simulink model "MotorModelDiscrete"  (R2019b)
settings: Solver=FixedStepAuto  StartTime=0.0  StopTime=8  FixedStep=Ts  RelTol=1e-3
undefined symbols (not defined in the file or in its folder): Discrete, motor, sensitivity_arduino, sigbuilder_block, Time, Ts
libraries: simulink x1, ctrlSharedLib x1, cstblocks x1, dspstat3 x1
settings Model: EnablePacing=on  Creator=miche  LastModifiedBy=AndreaCalegari

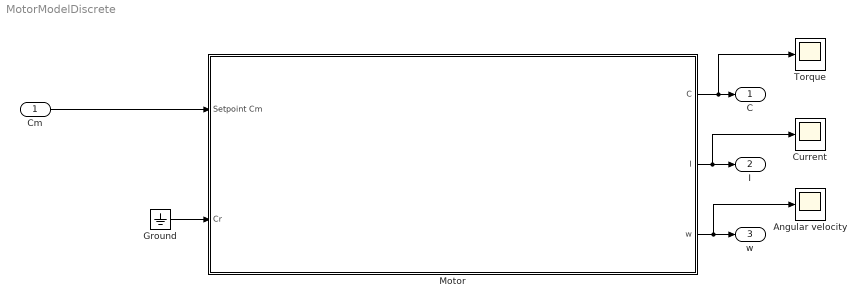
== system MotorModelDiscrete ==
  Cm : Inport
  Angular velocity : Scope
  Current : Scope
  Ground : Ground
  "Motor " : Subsystem
  Torque : Scope
  C : Outport
  I : Outport  Port=2
  w : Outport  Port=3
  wires:
  "Motor "/1("C ") -> Torque/1, C/1
  "Motor "/2("I ") -> Current/1, I/1
  "Motor "/3(w) -> Angular velocity/1, w/1
  Ground/1 -> "Motor "/2(Cr)
  Cm/1 -> "Motor "/1(Setpoint Cm)

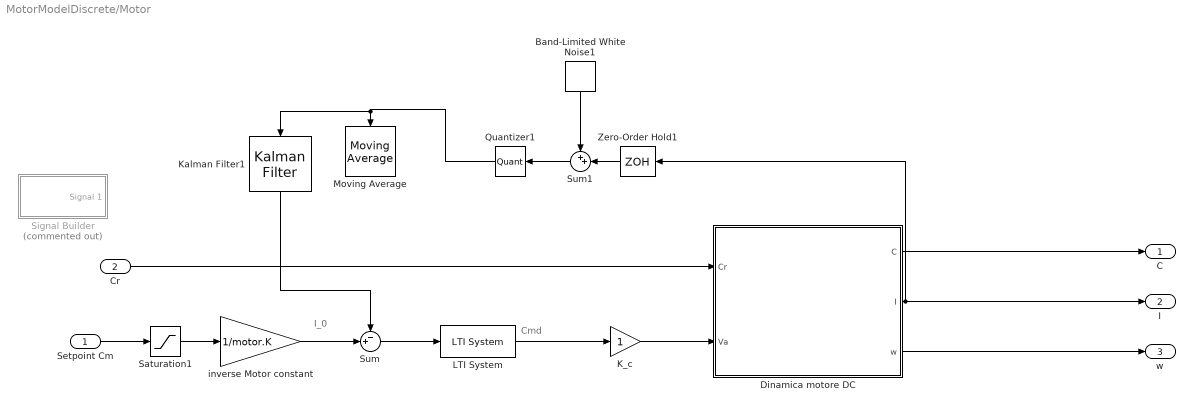
== system MotorModelDiscrete/Motor  ==
  note: Cmd
  note: I_0
  Setpoint Cm : Inport
  Cr : Inport  Port=2
  Band-Limited White Noise1 : simulink/Sources/Band-Limited White Noise  Cov=[0.00000001]  Ts=0.001  seed=[23341]
  Dinamica motore DC : Subsystem
  K_c : Gain
  Kalman Filter1 : ctrlSharedLib/Kalman Filter  TimeDomain=Discrete-Time  UseCurrentEstimator=on  ModelSource=Individual A, B, C, D matrices  ModelSourceVariable=ss(0.95,1,1,0,1)  A=0.999  B=1  C=1  D=0  NumberOfStates=1  NumberOfInputs=1  NumberOfOutputs=1  InitialEstimateSource=Dialog  X0=0  P0=10  UseK=off  UseGH=off  NumberOfProcessNoiseInputs=1  G=1  TimeInvariantG=on  H=0  TimeInvariantH=on  Q=0.1  TimeInvariantQ=on  R=1  TimeInvariantR=on  N=0  TimeInvariantN=on  AddInputPort=off  AddEnablePort=off  OutputEstimatedY=off  OutputP=off  Ts=-1
      settings: SourceProductBaseCode=CT
  LTI System : cstblocks/LTI System  sys=currentClosedLoop.PI_regulator_discrete  IC=[]
  Moving Average : dspstat3/Moving Average  Method=Sliding window  ForgettingFactorPort=off  SpecifyWindowLength=on  WindowLength=200  ForgettingFactor=0.9  SimulateUsing=Code generation
  Quantizer1 : Quantizer  QuantizationInterval=1/sensitivity_arduino
  Saturation1 : Saturate  UpperLimit=motor.Cmax  LowerLimit=-motor.Cmax
  Signal Builder : Subsystem  Tag=STV Subsys  Commented=on  LoadFcn=sigbuilder_block('load');  StartFcn=sigbuilder_block('start');  StopFcn=sigbuilder_block('stop');  ClipboardFcn=sigbuilder_block('clipboard');  mask(Sigbuilder block){tuvar=[0:10]}
      mask help: Simulink:masks:SigbuilderBlock_MD
      mask init:
      | if ~strcmp(get_param(bdroot(gcbh),'SimulationStatus'),'stopped') tuvar = sigbuilder_block('maskInit'); end
      settings: CopyFcn=sigbuilder_block('copy');  DeleteFcn=sigbuilder_block('delete');  ModelCloseFcn=sigbuilder_block('modelClose');  PreSaveFcn=sigbuilder_block('preSave');  PauseFcn=sigbuilder_block('pause');  ContinueFcn=sigbuilder_block('continue');  NameChangeFcn=sigbuilder_block('namechange');  OpenFcn=sigbuilder_block('open',[440.25 156.75 544.5 355.5 ]);  CloseFcn=sigbuilder_block('close');
      mask Display: plot(0, 0, 100, 100,[2, 2, 32, 32, 2], [68, 8, 8, 68, 68],[32, 2], [38, 38], [32, 19, 2],[53, 60, 44], [32, 17, 17, 2],[16, 16, 31, 31]);txt = getActiveGroup(gcbh);text(2, 100, txt,'verticalAlignment', 'top');
  Sum : Sum  Inputs=-+|
  Sum1 : Sum  Inputs=++|
  Zero-Order Hold1 : ZeroOrderHold  SampleTime=Ts
  inverse Motor constant : Gain  Gain=1/motor.K
  "C " : Outport
  "I " : Outport  Port=2
  w : Outport  Port=3
  wires:
  inverse Motor constant/1 -> Sum/2
  Setpoint Cm/1 -> Saturation1/1
  Cr/1 -> Dinamica motore DC/1(Cr)
  K_c/1 -> Dinamica motore DC/2(Va)
  Dinamica motore DC/1(C) -> "C "/1
  Dinamica motore DC/3(w) -> w/1
  Quantizer1/1 -> Kalman Filter1/1, Moving Average/1
  Dinamica motore DC/2(I) -> Zero-Order Hold1/1, "I "/1
  Band-Limited White Noise1/1 -> Sum1/1
  Zero-Order Hold1/1 -> Sum1/2
  Sum1/1 -> Quantizer1/1
  Sum/1 -> LTI System/1
  LTI System/1 -> K_c/1
  Saturation1/1 -> inverse Motor constant/1
  Kalman Filter1/1 -> Sum/1

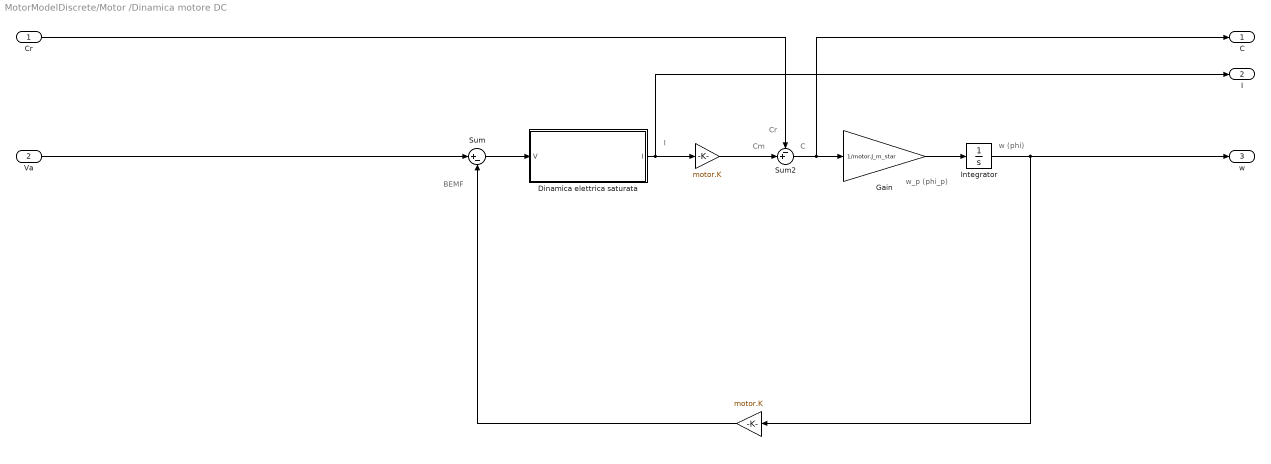
== system MotorModelDiscrete/Motor /Dinamica motore DC ==
  note: w (phi)
  note: C
  note: I
  note: Cm
  note: Cr
  note: w_p (phi_p)
  note: BEMF
  Cr : Inport
  Va : Inport  Port=2
  " " : Gain  Gain=motor.K
  " " : Gain  Gain=motor.K
  "Dinamica elettrica saturata " : Subsystem
  Gain : Gain  Gain=1/motor.J_m_star
  Integrator : Integrator
  Sum : Sum  Inputs=|+-
  Sum2 : Sum  Inputs=-+|
  C : Outport
  I : Outport  Port=2
  w : Outport  Port=3
  wires:
  " "/1 -> Sum2/2
  Sum2/1 -> Gain/1, C/1
  Integrator/1 -> " "/1, w/1
  "Dinamica elettrica saturata "/1(I) -> I/1, " "/1
  Cr/1 -> Sum2/1
  " "/1 -> Sum/2
  Va/1 -> Sum/1
  Sum/1 -> "Dinamica elettrica saturata "/1(V)
  Gain/1 -> Integrator/1

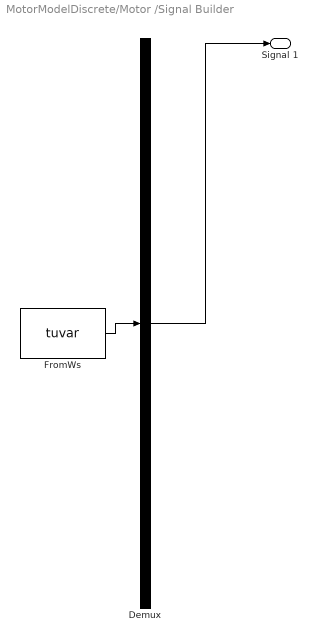
== system MotorModelDiscrete/Motor /Signal Builder ==
  Demux : Demux  Tag=STV Demux  Outputs=1
  FromWs : FromWorkspace  Tag=STV FromWs  VariableName=tuvar  SampleTime=0
      SigBuilderData=|
      | common.afterFinalStr = 'Extrapolate'
      | common.sampleTime = 0
      | dataSet.timeRange = [0 10]
      | dataSet.name = 'Group 1'
      | sbobj.Groups.Name = 'Group 1'
      | sbobj.Groups.Signals.Name = 'Signal 1'
      | sbobj.Groups.Signals.XData = [0 5 5 10]
      | sbobj.Groups.Signals.YData = [5 5 -5 -5]
  Signal 1 : Outport  Tag=STV Outport
  wires:
  Demux/1 -> Signal 1/1
  FromWs/1 -> Demux/1

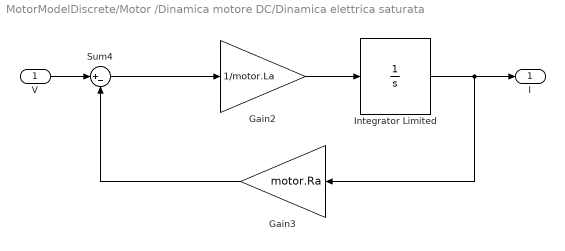
== system MotorModelDiscrete/Motor /Dinamica motore DC/Dinamica elettrica saturata  ==
  V : Inport
  Gain2 : Gain  Gain=1/motor.La
  Gain3 : Gain  Gain=motor.Ra
  Integrator Limited : Integrator  LimitOutput=on  UpperSaturationLimit=motor.Imax  LowerSaturationLimit=-motor.Imax
  Sum4 : Sum  Inputs=|+-
  I : Outport
  wires:
  Gain3/1 -> Sum4/2
  Sum4/1 -> Gain2/1
  Gain2/1 -> Integrator Limited/1
  Integrator Limited/1 -> I/1, Gain3/1
  V/1 -> Sum4/1
